simulink model "Sistema2Orden"  (R2015a)
settings: Solver=ode45  StartTime=0.0  StopTime=20  RelTol=1e-3
undefined symbols (not defined in the file or in its folder): C, L, R
settings Model: Creator=casa  LastModifiedBy=casa

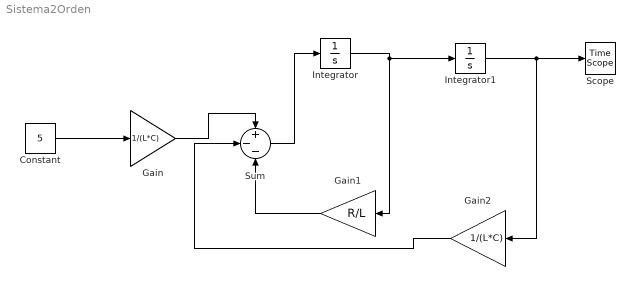
== system Sistema2Orden ==
  Constant : Constant  Value=5
  Gain : Gain  Gain=1/(L*C)
  Gain1 : Gain  Gain=R/L
  Gain2 : Gain  Gain=1/(L*C)
  Integrator : Integrator
  Integrator1 : Integrator
  Scope : TimeScope
  Sum : Sum  Inputs=+--
  wires:
  Constant/1 -> Gain/1
  Gain/1 -> Sum/1
  Sum/1 -> Integrator/1
  Integrator/1 -> Integrator1/1, Gain1/1
  Gain1/1 -> Sum/3
  Gain2/1 -> Sum/2
  Integrator1/1 -> Scope/1, Gain2/1
